simulink model "pmsm_dq_svpwm_cascade"  (R2025b)
settings: Solver=FixedStepDiscrete  StartTime=0.0  StopTime=4  FixedStep=5e-05  RelTol=1e-3
model workspace (MAT data in the model file):
  pmsm.Vdc = 36
  pmsm.Ts = 5e-05
  pmsm.StopTime = 4
  pmsm.StepTime = 0.02
  pmsm.PositionStep = 1
  pmsm.LoadStepTime = 1.8
  pmsm.LoadTorqueInitial = 0
  pmsm.Rs = 0.6
  pmsm.Ld = 0.00082
  pmsm.Lq = 0.00082
  pmsm.PolePairs = 14
  pmsm.KvRpmPerVolt = 6.71
  pmsm.MaxSpeedRpm = 1500
  pmsm.KvAssumption = "raw user value; PsiF is estimated from Vdc and MaxSpeedRpm"
  pmsm.PsiF = 0.00945135249295
  pmsm.Kt = 0.198478402352
  pmsm.GearStage1Ratio = 3.71428571428
  pmsm.GearStage2Ratio = 14
  pmsm.GearTotalRatio = 51.9999999999
  pmsm.GearEfficiency = 1
  pmsm.OutputMaxSpeedRpm = 28.8461538462
  pmsm.RatedTorqueMotor = 0.7
  pmsm.StallTorqueMotor = 2.2
  pmsm.RatedTorqueOutput = 36.3999999999
  pmsm.StallTorqueOutput = 114.4
  pmsm.LoadTorqueStallFraction = 0.9
  pmsm.LoadTorqueFinal = 102.96
  pmsm.RatedCurrentFromTorque = 3.52683209712
  pmsm.StallCurrentFromTorque = 11.0843294481
  pmsm.J = 8e-05
  pmsm.B = 0.0001
  pmsm.RatedCurrent = 3.8
  pmsm.PeakCurrent = 19.5
  pmsm.IdRef = 0
  pmsm.IqLimit = 11.0843294481
  pmsm.OmegaLimit = 3.02076216692
  pmsm.VoltageLimit = 20.7846096908
  pmsm.KpPosition = 2
  pmsm.KiPosition = 0
  pmsm.KpSpeed = 0.08
  pmsm.KiSpeed = 1
  pmsm.KpCurrent = 1.23
  pmsm.KiCurrent = 900
settings Model: Creator=fluoroantimonic_acid  LastModifiedBy=fluoroantimonic_acid
settings DataIOCC: SaveOutput=off

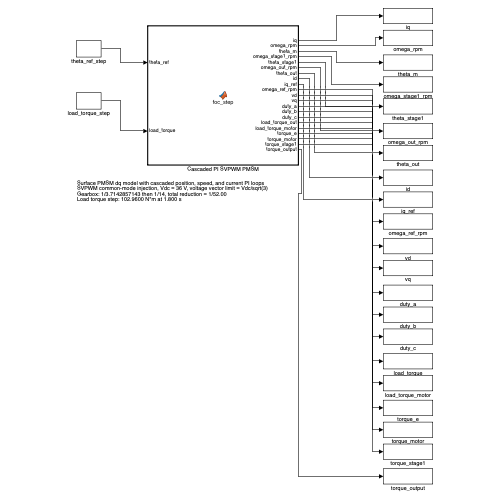
[thumbnail: Simulink's stored preview of the top-level diagram]
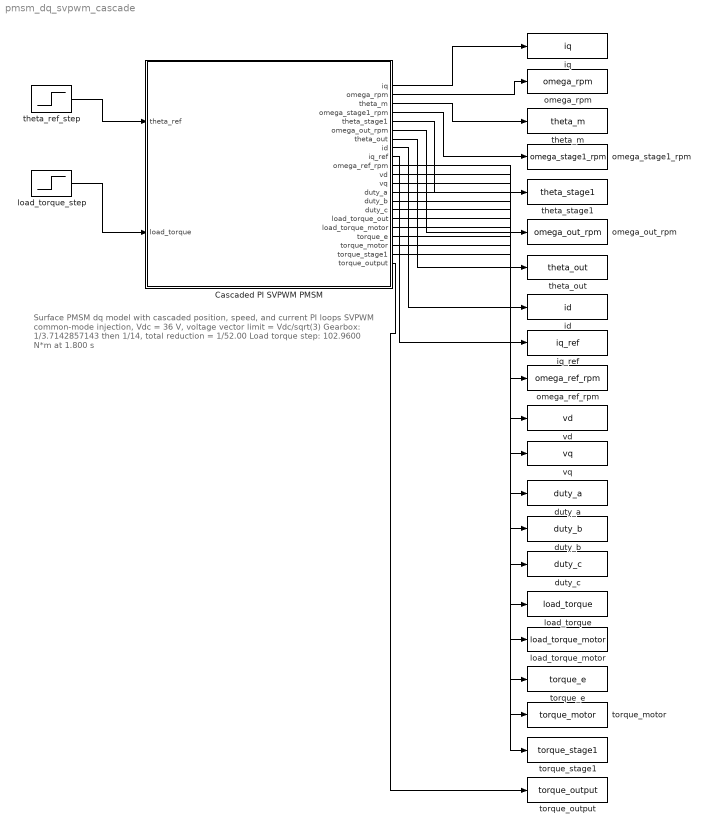
== system pmsm_dq_svpwm_cascade ==
  note: Surface PMSM dq model with cascaded position, speed, and current PI loops
      | SVPWM common-mode injection, Vdc = 36 V, voltage vector limit = Vdc/sqrt(3)
      | Gearbox: 1/3.7142857143 then 1/14, total reduction = 1/52.00
      | Load torque step: 102.9600 N*m at 1.800 s
  Cascaded PI SVPWM PMSM : MATLAB Function  TreatAsAtomicUnit=on
  duty_a : ToWorkspace  VariableName=duty_a  SaveFormat=Timeseries  SampleTime=-1
  duty_b : ToWorkspace  VariableName=duty_b  SaveFormat=Timeseries  SampleTime=-1
  duty_c : ToWorkspace  VariableName=duty_c  SaveFormat=Timeseries  SampleTime=-1
  id : ToWorkspace  VariableName=id  SaveFormat=Timeseries  SampleTime=-1
  iq : ToWorkspace  VariableName=iq  SaveFormat=Timeseries  SampleTime=-1
  iq_ref : ToWorkspace  VariableName=iq_ref  SaveFormat=Timeseries  SampleTime=-1
  load_torque : ToWorkspace  VariableName=load_torque  SaveFormat=Timeseries  SampleTime=-1
  load_torque_motor : ToWorkspace  VariableName=load_torque_motor  SaveFormat=Timeseries  SampleTime=-1
  load_torque_step : Step  Time=1.8  After=102.96  SampleTime=5e-05
  omega_out_rpm : ToWorkspace  VariableName=omega_out_rpm  SaveFormat=Timeseries  SampleTime=-1
  omega_ref_rpm : ToWorkspace  VariableName=omega_ref_rpm  SaveFormat=Timeseries  SampleTime=-1
  omega_rpm : ToWorkspace  VariableName=omega_rpm  SaveFormat=Timeseries  SampleTime=-1
  omega_stage1_rpm : ToWorkspace  VariableName=omega_stage1_rpm  SaveFormat=Timeseries  SampleTime=-1
  theta_m : ToWorkspace  VariableName=theta_m  SaveFormat=Timeseries  SampleTime=-1
  theta_out : ToWorkspace  VariableName=theta_out  SaveFormat=Timeseries  SampleTime=-1
  theta_ref_step : Step  Time=0.02  SampleTime=5e-05
  theta_stage1 : ToWorkspace  VariableName=theta_stage1  SaveFormat=Timeseries  SampleTime=-1
  torque_e : ToWorkspace  VariableName=torque_e  SaveFormat=Timeseries  SampleTime=-1
  torque_motor : ToWorkspace  VariableName=torque_motor  SaveFormat=Timeseries  SampleTime=-1
  torque_output : ToWorkspace  VariableName=torque_output  SaveFormat=Timeseries  SampleTime=-1
  torque_stage1 : ToWorkspace  VariableName=torque_stage1  SaveFormat=Timeseries  SampleTime=-1
  vd : ToWorkspace  VariableName=vd  SaveFormat=Timeseries  SampleTime=-1
  vq : ToWorkspace  VariableName=vq  SaveFormat=Timeseries  SampleTime=-1
  wires:
  theta_ref_step/1 -> Cascaded PI SVPWM PMSM/1(theta_ref)
  load_torque_step/1 -> Cascaded PI SVPWM PMSM/2(load_torque)
  Cascaded PI SVPWM PMSM/1(iq) -> iq/1
  Cascaded PI SVPWM PMSM/2(omega_rpm) -> omega_rpm/1
  Cascaded PI SVPWM PMSM/3(theta_m) -> theta_m/1
  Cascaded PI SVPWM PMSM/4(omega_stage1_rpm) -> omega_stage1_rpm/1
  Cascaded PI SVPWM PMSM/5(theta_stage1) -> theta_stage1/1
  Cascaded PI SVPWM PMSM/6(omega_out_rpm) -> omega_out_rpm/1
  Cascaded PI SVPWM PMSM/7(theta_out) -> theta_out/1
  Cascaded PI SVPWM PMSM/8(id) -> id/1
  Cascaded PI SVPWM PMSM/9(iq_ref) -> iq_ref/1
  Cascaded PI SVPWM PMSM/10(omega_ref_rpm) -> omega_ref_rpm/1
  Cascaded PI SVPWM PMSM/11(vd) -> vd/1
  Cascaded PI SVPWM PMSM/12(vq) -> vq/1
  Cascaded PI SVPWM PMSM/13(duty_a) -> duty_a/1
  Cascaded PI SVPWM PMSM/14(duty_b) -> duty_b/1
  Cascaded PI SVPWM PMSM/15(duty_c) -> duty_c/1
  Cascaded PI SVPWM PMSM/16(load_torque_out) -> load_torque/1
  Cascaded PI SVPWM PMSM/17(load_torque_motor) -> load_torque_motor/1
  Cascaded PI SVPWM PMSM/18(torque_e) -> torque_e/1
  Cascaded PI SVPWM PMSM/19(torque_motor) -> torque_motor/1
  Cascaded PI SVPWM PMSM/20(torque_stage1) -> torque_stage1/1
  Cascaded PI SVPWM PMSM/21(torque_output) -> torque_output/1

== matlab function pmsm_dq_svpwm_cascade/Cascaded PI SVPWM PMSM ==
  data: theta_ref input; iq output; load_torque input; omega_rpm output; theta_m output; omega_stage1_rpm output; theta_stage1 output; omega_out_rpm output; theta_out output; id output; iq_ref output; omega_ref_rpm output; vd output; vq output; duty_a output; duty_b output; duty_c output; load_torque_out output; load_torque_motor output; torque_e output; torque_motor output; torque_stage1 output; torque_output output
function [iq, omega_rpm, theta_m, omega_stage1_rpm, theta_stage1, omega_out_rpm, theta_out, id, iq_ref, omega_ref_rpm, vd, vq, duty_a, duty_b, duty_c, load_torque_out, load_torque_motor, torque_e, torque_motor, torque_stage1, torque_output] = foc_step(theta_ref, load_torque)
%#codegen
persistent id_state iq_state omega_state theta_state int_pos int_speed int_d int_q
if isempty(id_state)
    id_state = 0;
    iq_state = 0;
    omega_state = 0;
    theta_state = 0;
    int_pos = 0;
    int_speed = 0;
    int_d = 0;
    int_q = 0;
end

Ts = 5.0000000000000002e-05;
Vdc = 36;
Rs = 0.59999999999999998;
Ld = 0.00081999999999999998;
Lq = 0.00081999999999999998;
psi_f = 0.0094513524929450057;
pole_pairs = 14;
J = 8.0000000000000007e-05;
B = 0.0001;
max_omega_motor = 157.07963267948966;
gear_stage1 = 3.7142857142799999;
gear_total = 51.99999999992;
gear_efficiency = 1;
id_ref = 0;
iq_limit = 11.084329448098;
phase_current_limit = 19.5;
omega_limit = 3.0207621669179101;
voltage_limit = Vdc / sqrt(3);
kp_pos = 2;
ki_pos = 0;
kp_speed = 0.080000000000000002;
ki_speed = 1;
kp_current = 1.23;
ki_current = 900;

theta_out_state = theta_state / gear_total;
omega_out_state = omega_state / gear_total;
theta_error = theta_ref - theta_out_state;
[omega_ref, int_pos] = pi_limit(theta_error, int_pos, kp_pos, ki_pos, Ts, -omega_limit, omega_limit);

speed_error = omega_ref - omega_out_state;
[iq_ref, int_speed] = pi_limit(speed_error, int_speed, kp_speed, ki_speed, Ts, -iq_limit, iq_limit);

omega_e = pole_pairs * omega_state;
id_error = id_ref - id_state;
iq_error = iq_ref - iq_state;

[vd_pi, int_d] = pi_limit(id_error, int_d, kp_current, ki_current, Ts, -voltage_limit, voltage_limit);
[vq_pi, int_q] = pi_limit(iq_error, int_q, kp_current, ki_current, Ts, -voltage_limit, voltage_limit);

vd_ff = -omega_e * Lq * iq_state;
vq_ff = omega_e * (Ld * id_state + psi_f);
vd_cmd = vd_pi + vd_ff;
vq_cmd = vq_pi + vq_ff;
[vd, vq] = limit_vector(vd_cmd, vq_cmd, voltage_limit);

did = (vd - Rs * id_state + omega_e * Lq * iq_state) / Ld;
diq = (vq - Rs * iq_state - omega_e * (Ld * id_state + psi_f)) / Lq;
torque_e = 1.5 * pole_pairs * (psi_f * iq_state + (Ld - Lq) * id_state * iq_state);
load_torque_motor = load_torque / (gear_total * gear_efficiency);
domega = (torque_e - load_torque_motor - B * omega_state) / J;

id_state = saturate(id_state + Ts * did, -phase_current_limit, phase_current_limit);
iq_state = saturate(iq_state + Ts * diq, -iq_limit, iq_limit);
omega_state = saturate(omega_state + Ts * domega, -max_omega_motor, max_omega_motor);
theta_state = theta_state + Ts * omega_state;

[duty_a, duty_b, duty_c] = svpwm_duty(vd, vq, theta_state, pole_pairs, Vdc);

id = id_state;
iq = iq_state;
theta_m = theta_state;
omega_rpm = omega_state * 60 / (2 * pi);
theta_stage1 = theta_state / gear_stage1;
omega_stage1_rpm = omega_rpm / gear_stage1;
theta_out = theta_state / gear_total;
omega_out_rpm = omega_rpm / gear_total;
omega_ref_rpm = omega_ref * 60 / (2 * pi);
load_torque_out = load_torque;
torque_motor = torque_e;
torque_stage1 = torque_motor * gear_stage1 * gear_efficiency;
torque_output = torque_motor * gear_total * gear_efficiency;
end

function [u, integrator] = pi_limit(error, integrator, kp, ki, Ts, min_value, max_value)
candidate_integrator = integrator + ki * Ts * error;
raw = kp * error + candidate_integrator;
u_candidate = saturate(raw, min_value, max_value);
if raw == u_candidate || (raw > max_value && error < 0) || (raw < min_value && error > 0)
    integrator = candidate_integrator;
end
u = saturate(kp * error + integrator, min_value, max_value);
end

function [d_axis, q_axis] = limit_vector(d_axis, q_axis, limit_value)
magnitude = sqrt(d_axis * d_axis + q_axis * q_axis);
if magnitude > limit_value && magnitude > 0
    scale = limit_value / magnitude;
    d_axis = d_axis * scale;
    q_axis = q_axis * scale;
end
end

function value = saturate(value, min_value, max_value)
if value > max_value
    value = max_value;
elseif value < min_value
    value = min_value;
end
end

function [duty_a, duty_b, duty_c] = svpwm_duty(vd, vq, theta_m, pole_pairs, Vdc)
theta_e = pole_pairs * theta_m;
cos_e = cos(theta_e);
sin_e = sin(theta_e);
v_alpha = cos_e * vd - sin_e * vq;
v_beta = sin_e * vd + cos_e * vq;

v_a = v_alpha;
v_b = -0.5 * v_alpha + sqrt(3) * 0.5 * v_beta;
v_c = -0.5 * v_alpha - sqrt(3) * 0.5 * v_beta;

v_max = max(v_a, max(v_b, v_c));
v_min = min(v_a, min(v_b, v_c));
v_zero = -0.5 * (v_max + v_min);

duty_a = saturate(0.5 + (v_a + v_zero) / Vdc, 0, 1);
duty_b = saturate(0.5 + (v_b + v_zero) / Vdc, 0, 1);
duty_c = saturate(0.5 + (v_c + v_zero) / Vdc, 0, 1);
end
